simulink model "RoboticArm"  (R2023b)
settings: Solver=ode23t  StartTime=0.0  StopTime=100  RelTol=1e-3
model workspace: external: MATLAB File D:\Projects\RoboticArm\RoboticArm_DataFile1.m (data not in the file)
undefined symbols (not defined in the file or in its folder): dfdbk, dFilt, nfdbk, nFilt, smiData, ST, X, Y, Z
libraries: sm_lib x180, fl_lib x129, nesl_utility x69, ee_lib x39, slpidlib x25, simulink x18, SignalEditorBlockLib x1
(part 1 of 7)
settings Model: Creator=ASUS  LastModifiedBy=ASUS

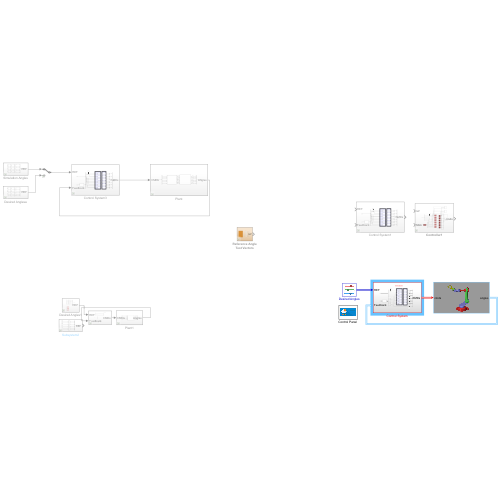
[thumbnail: Simulink's stored preview of the top-level diagram]
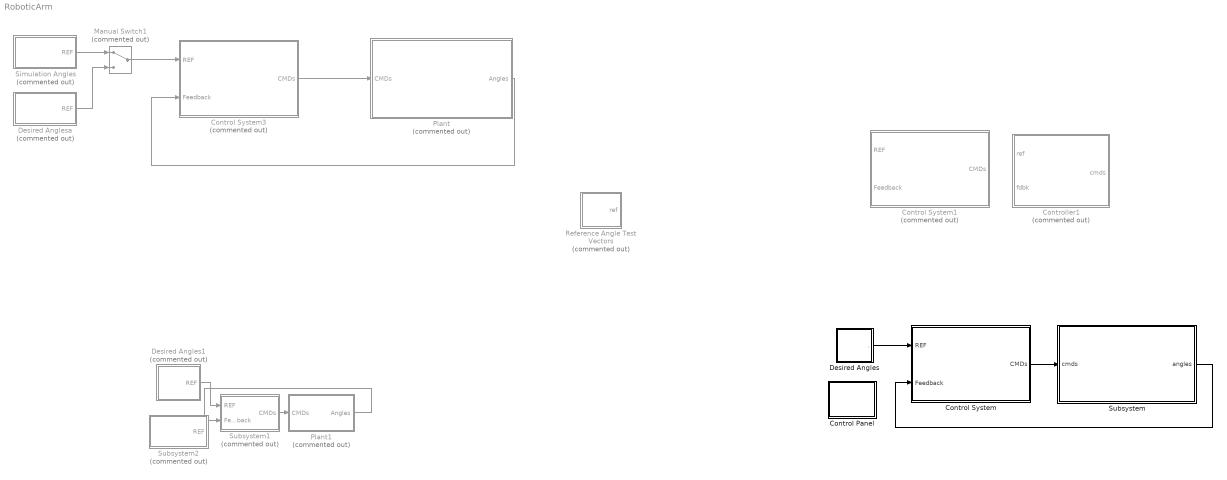
== system RoboticArm ==
  "Control Panel " : Subsystem
      mask Display: image('OIP (1).jpg');
  Control System : Subsystem
  Control System1 : Subsystem  Commented=on
  Control System3 : Subsystem  Commented=on
  Controller1 : Subsystem  Commented=on
  Desired Angles : Subsystem
      mask Display: image('reference.webp');
  Desired Angles1 : Subsystem  Commented=on
  Desired Anglesa : Subsystem  Commented=on
  Manual Switch1 : ManualSwitch  Commented=on
  Plant : Subsystem  Commented=on
  Plant1 : Subsystem  Commented=on
  Reference Angle Test Vectors : Subsystem  Commented=on
  Simulation Angles : Subsystem  Commented=on
  Subsystem : Subsystem
      mask Display: image('Screenshot 2024-04-15 220619.png');
  Subsystem1 : Subsystem  Commented=on
  Subsystem2 : Subsystem  Commented=on
  wires:
  Plant/1(Angles) -> Control System3/2(Feedback)
  Control System3/1(CMDs) -> Plant/1(CMDs)
  Subsystem1/1(CMDs) -> Plant1/1(CMDs)
  Plant1/1(Angles) -> Subsystem1/2(Feedback)
  Desired Angles1/1(REF) -> Subsystem1/1(REF)
  Desired Angles/1(.) -> Control System/1(REF)
  Subsystem/1(angles) -> Control System/2(Feedback)
  Control System/1(CMDs) -> Subsystem/1(cmds)
  Simulation Angles/1(REF) -> Manual Switch1/1
  Manual Switch1/1 -> Control System3/1(REF)
  Desired Anglesa/1(REF) -> Manual Switch1/2

== system RoboticArm/Control Panel  ==
  "Bicep " : Subsystem
      mask Display: image('Screenshot 2024-04-15 210704.png');
  Forearm : Subsystem
      mask Display: image('Screenshot 2024-04-15 210823.png');
  Gripper : Subsystem
      mask Display: image('Screenshot 2024-04-15 212833.png');
  Gripper base : Subsystem
      mask Display: image('Screenshot 2024-04-15 211030.png');
  Hand : Subsystem
      mask Display: image('Screenshot 2024-04-15 210946.png');
  Slider{,1..5} (6 alike) : SliderBlock  ScaleMin=-90  ScaleMax=90
  Slider6 : SliderBlock  ScaleMin=100  ScaleMax=140
  Turntable : Subsystem
      mask Display: image('Screenshot 2024-04-15 210633.png');
  Wrist : Subsystem
      mask Display: image('Screenshot 2024-04-15 210901.png');

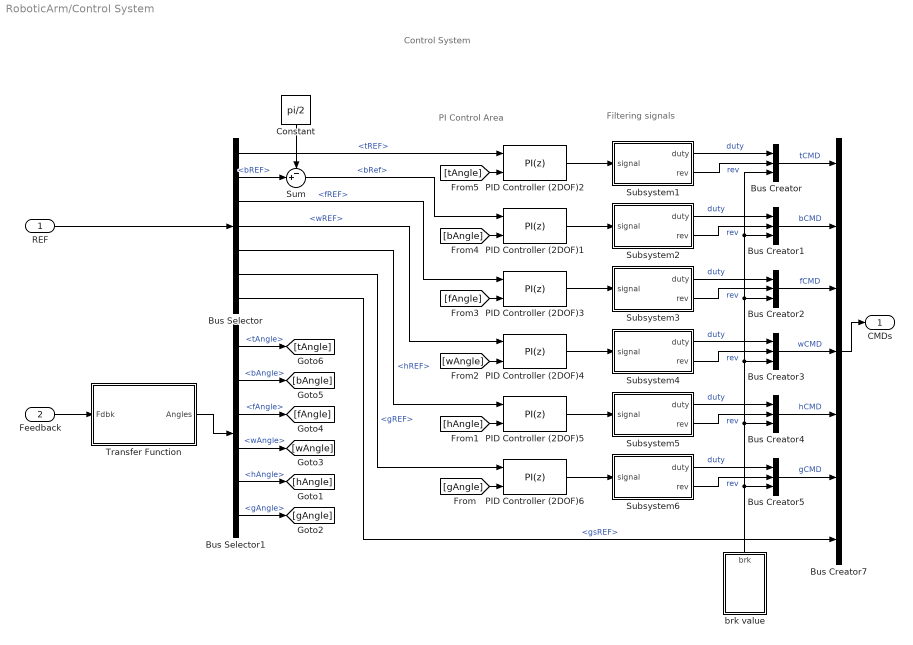
== system RoboticArm/Control System ==
  note: Control System
  note: PI Control Area
  note: Filtering signals
  REF : Inport
  Feedback : Inport  Port=2
  Bus Creator{,1..5} (6 alike) : BusCreator  Inputs=3
  Bus Creator7 : BusCreator  Inputs=7
  Bus Selector : BusSelector  OutputSignals=tREF,bREF,fREF,wREF,hREF,gREF,gsREF
  Bus Selector1 : BusSelector  OutputSignals=tAngle,bAngle,fAngle,wAngle,hAngle,gAngle
  Constant : Constant  Value=pi/2
  PID Controller (2DOF)1 : slpidlib/PID Controller (2DOF)  Controller=PI  Form=Parallel  TimeDomain=Discrete-time  UseExternalTs=off  SampleTime=ST  IntegratorMethod=Forward Euler  FilterMethod=Forward Euler  ControllerParametersSource=internal  P=6  I=3  UseKiTs=off  D=0.001  N=100  UseFilter=on  b=1  c=1  TunerSelectOption=Frequency Response Based  InitialConditionSource=internal  InitialConditionForIntegrator=0  InitialConditionForFilter=0  DifferentiatorICPrevScaledInput=0  ExternalReset=none  TrackingMode=off  Kt=1  LimitOutput=off  SatLimitsSource=internal  UpperSaturationLimit=inf  LowerSaturationLimit=-inf  LinearizeAsGain=on  AntiWindupMode=none  Kb=1  LimitIntegrator=off  UpperIntegratorSaturationLimit=inf  LowerIntegratorSaturationLimit=-inf  POutMin=[]  POutMax=[]  IOutMin=[]  IOutMax=[]  DOutMin=[]  DOutMax=[]  NOutMin=[]  NOutMax=[]  bOutMin=[]  bOutMax=[]  cOutMin=[]  cOutMax=[]  SumOutMin=[]  SumOutMax=[]  SaturationOutMin=[]  SaturationOutMax=[]  PParamMin=[]  PParamMax=[]  IParamMin=[]  IParamMax=[]  DParamMin=[]  DParamMax=[]  NParamMin=[]  NParamMax=[]  bParamMin=[]  bParamMax=[]  cParamMin=[]  cParamMax=[]  KbParamMin=[]  KbParamMax=[]  KtParamMin=[]  KtParamMax=[]  KbOutMin=[]  KbOutMax=[]  KtOutMin=[]  KtOutMax=[]  IntegratorOutMin=[]  IntegratorOutMax=[]  FilterOutMin=[]  FilterOutMax=[]  SumI1OutMin=[]  SumI1OutMax=[]  SumI2OutMin=[]  SumI2OutMax=[]  SumI3OutMin=[]  SumI3OutMax=[]  SumI4OutMin=[]  SumI4OutMax=[]  SumDOutMin=[]  SumDOutMax=[]  Sum1OutMin=[]  Sum1OutMax=[]  Sum2OutMin=[]  Sum2OutMax=[]  Sum3OutMin=[]  Sum3OutMax=[]  DifferentiatorOutMin=[]  DifferentiatorOutMax=[]  FilterDiffOutCoefMin=[]  FilterDiffOutCoefMax=[]  ReciprocalOutMin=[]  ReciprocalOutMax=[]  SumDenOutMin=[]  SumDenOutMax=[]  SumNumOutMin=[]  SumNumOutMax=[]  DivideOutMin=[]  DivideOutMax=[]  UdiffTsProdOutMin=[]  UdiffTsProdOutMax=[]  NTsProdOutMin=[]  NTsProdOutMax=[]  UintegralTsProdOutMin=[]  UintegralTsProdOutMax=[]  UngainTsProdOutMin=[]  UngainTsProdOutMax=[]  ClampingZeroOutDataTypeStr=Inherit: Inherit via back propagation  ClampingZeroOutMin=[]  ClampingZeroOutMax=[]  FilterDenConstantOutDataTypeStr=Inherit: Inherit via back propagation  FilterDenConstantOutMin=[]  FilterDenConstantOutMax=[]  PCopyOutDataTypeStr=Inherit: Inherit via back propagation  PCopyOutMin=[]  PCopyOutMax=[]  NCopyOutDataTypeStr=Inherit: Inherit via back propagation  NCopyOutMin=[]  NCopyOutMax=[]  IntegratorContinuousStateAttributes=''  IntegratorStateMustResolveToSignalObject=off  IntegratorRTWStateStorageClass=Auto  FilterContinuousStateAttributes=''  FilterStateMustResolveToSignalObject=off  FilterRTWStateStorageClass=Auto  ParallelPVariant=InternalParameters  IdealPVariant=Disabled  IVariant=InternalParameters  DVariant=Disabled  bVariant=InternalParameters  cVariant=Disabled  IntegratorVariant=Discrete  SatVariant=Disabled  AWVariant=Passthrough  PCopyVariant=Disabled  TRVariant=Disabled  FdbkBlocksVariant=Forward  IdealPFdbkVariant=Disabled  SatFdbkVariant=Disabled  DerivativeFilterVariant=Disabled  NVariant=Disabled  NCopyVariant=Disabled_SignalSpec  FilterICVariant=Disabled  IntegratorICVariant=InternalICs  ExternalResetVariant=Disabled  TRSumVariant=Passthrough  SumFdbkVariant=Disabled  SumVariant=Sum_PI  TsampFilterVariant=InternalTs  TsampNgainVariant=Passthrough  TsampIntegralVariant=Disabled_SignalSpec  ExternalSaturationOutDataTypeStr=Inherit: Same as second input
  PID Controller (2DOF){2,4..6} (4 alike) : slpidlib/PID Controller (2DOF)  Controller=PI  Form=Parallel  TimeDomain=Discrete-time  UseExternalTs=off  SampleTime=ST  IntegratorMethod=Forward Euler  FilterMethod=Forward Euler  ControllerParametersSource=internal  P=3  I=3  UseKiTs=off  D=0.001  N=100  UseFilter=on  b=1  c=1  TunerSelectOption=Frequency Response Based  InitialConditionSource=internal  InitialConditionForIntegrator=0  InitialConditionForFilter=0  DifferentiatorICPrevScaledInput=0  ExternalReset=none  TrackingMode=off  Kt=1  LimitOutput=off  SatLimitsSource=internal  UpperSaturationLimit=inf  LowerSaturationLimit=-inf  LinearizeAsGain=on  AntiWindupMode=none  Kb=1  LimitIntegrator=off  UpperIntegratorSaturationLimit=inf  LowerIntegratorSaturationLimit=-inf  POutMin=[]  POutMax=[]  IOutMin=[]  IOutMax=[]  DOutMin=[]  DOutMax=[]  NOutMin=[]  NOutMax=[]  bOutMin=[]  bOutMax=[]  cOutMin=[]  cOutMax=[]  SumOutMin=[]  SumOutMax=[]  SaturationOutMin=[]  SaturationOutMax=[]  PParamMin=[]  PParamMax=[]  IParamMin=[]  IParamMax=[]  DParamMin=[]  DParamMax=[]  NParamMin=[]  NParamMax=[]  bParamMin=[]  bParamMax=[]  cParamMin=[]  cParamMax=[]  KbParamMin=[]  KbParamMax=[]  KtParamMin=[]  KtParamMax=[]  KbOutMin=[]  KbOutMax=[]  KtOutMin=[]  KtOutMax=[]  IntegratorOutMin=[]  IntegratorOutMax=[]  FilterOutMin=[]  FilterOutMax=[]  SumI1OutMin=[]  SumI1OutMax=[]  SumI2OutMin=[]  SumI2OutMax=[]  SumI3OutMin=[]  SumI3OutMax=[]  SumI4OutMin=[]  SumI4OutMax=[]  SumDOutMin=[]  SumDOutMax=[]  Sum1OutMin=[]  Sum1OutMax=[]  Sum2OutMin=[]  Sum2OutMax=[]  Sum3OutMin=[]  Sum3OutMax=[]  DifferentiatorOutMin=[]  DifferentiatorOutMax=[]  FilterDiffOutCoefMin=[]  FilterDiffOutCoefMax=[]  ReciprocalOutMin=[]  ReciprocalOutMax=[]  SumDenOutMin=[]  SumDenOutMax=[]  SumNumOutMin=[]  SumNumOutMax=[]  DivideOutMin=[]  DivideOutMax=[]  UdiffTsProdOutMin=[]  UdiffTsProdOutMax=[]  NTsProdOutMin=[]  NTsProdOutMax=[]  UintegralTsProdOutMin=[]  UintegralTsProdOutMax=[]  UngainTsProdOutMin=[]  UngainTsProdOutMax=[]  ClampingZeroOutDataTypeStr=Inherit: Inherit via back propagation  ClampingZeroOutMin=[]  ClampingZeroOutMax=[]  FilterDenConstantOutDataTypeStr=Inherit: Inherit via back propagation  FilterDenConstantOutMin=[]  FilterDenConstantOutMax=[]  PCopyOutDataTypeStr=Inherit: Inherit via back propagation  PCopyOutMin=[]  PCopyOutMax=[]  NCopyOutDataTypeStr=Inherit: Inherit via back propagation  NCopyOutMin=[]  NCopyOutMax=[]  IntegratorContinuousStateAttributes=''  IntegratorStateMustResolveToSignalObject=off  IntegratorRTWStateStorageClass=Auto  FilterContinuousStateAttributes=''  FilterStateMustResolveToSignalObject=off  FilterRTWStateStorageClass=Auto  ParallelPVariant=InternalParameters  IdealPVariant=Disabled  IVariant=InternalParameters  DVariant=Disabled  bVariant=InternalParameters  cVariant=Disabled  IntegratorVariant=Discrete  SatVariant=Disabled  AWVariant=Passthrough  PCopyVariant=Disabled  TRVariant=Disabled  FdbkBlocksVariant=Forward  IdealPFdbkVariant=Disabled  SatFdbkVariant=Disabled  DerivativeFilterVariant=Disabled  NVariant=Disabled  NCopyVariant=Disabled_SignalSpec  FilterICVariant=Disabled  IntegratorICVariant=InternalICs  ExternalResetVariant=Disabled  TRSumVariant=Passthrough  SumFdbkVariant=Disabled  SumVariant=Sum_PI  TsampFilterVariant=InternalTs  TsampNgainVariant=Passthrough  TsampIntegralVariant=Disabled_SignalSpec  ExternalSaturationOutDataTypeStr=Inherit: Same as second input
  PID Controller (2DOF)3 : slpidlib/PID Controller (2DOF)  Controller=PI  Form=Parallel  TimeDomain=Discrete-time  UseExternalTs=off  SampleTime=ST  IntegratorMethod=Forward Euler  FilterMethod=Forward Euler  ControllerParametersSource=internal  P=6  I=3  UseKiTs=off  D=0.001  N=100  UseFilter=on  b=1  c=1  TunerSelectOption=Frequency Response Based  InitialConditionSource=internal  InitialConditionForIntegrator=0  InitialConditionForFilter=0  DifferentiatorICPrevScaledInput=0  ExternalReset=none  TrackingMode=off  Kt=1  LimitOutput=off  SatLimitsSource=internal  UpperSaturationLimit=inf  LowerSaturationLimit=-inf  LinearizeAsGain=on  AntiWindupMode=none  Kb=1  LimitIntegrator=off  UpperIntegratorSaturationLimit=inf  LowerIntegratorSaturationLimit=-inf  POutMin=[]  POutMax=[]  IOutMin=[]  IOutMax=[]  DOutMin=[]  DOutMax=[]  NOutMin=[]  NOutMax=[]  bOutMin=[]  bOutMax=[]  cOutMin=[]  cOutMax=[]  SumOutMin=[]  SumOutMax=[]  SaturationOutMin=[]  SaturationOutMax=[]  PParamMin=[]  PParamMax=[]  IParamMin=[]  IParamMax=[]  DParamMin=[]  DParamMax=[]  NParamMin=[]  NParamMax=[]  bParamMin=[]  bParamMax=[]  cParamMin=[]  cParamMax=[]  KbParamMin=[]  KbParamMax=[]  KtParamMin=[]  KtParamMax=[]  KbOutMin=[]  KbOutMax=[]  KtOutMin=[]  KtOutMax=[]  IntegratorOutMin=[]  IntegratorOutMax=[]  FilterOutMin=[]  FilterOutMax=[]  SumI1OutMin=[]  SumI1OutMax=[]  SumI2OutMin=[]  SumI2OutMax=[]  SumI3OutMin=[]  SumI3OutMax=[]  SumI4OutMin=[]  SumI4OutMax=[]  SumDOutMin=[]  SumDOutMax=[]  Sum1OutMin=[]  Sum1OutMax=[]  Sum2OutMin=[]  Sum2OutMax=[]  Sum3OutMin=[]  Sum3OutMax=[]  DifferentiatorOutMin=[]  DifferentiatorOutMax=[]  FilterDiffOutCoefMin=[]  FilterDiffOutCoefMax=[]  ReciprocalOutMin=[]  ReciprocalOutMax=[]  SumDenOutMin=[]  SumDenOutMax=[]  SumNumOutMin=[]  SumNumOutMax=[]  DivideOutMin=[]  DivideOutMax=[]  UdiffTsProdOutMin=[]  UdiffTsProdOutMax=[]  NTsProdOutMin=[]  NTsProdOutMax=[]  UintegralTsProdOutMin=[]  UintegralTsProdOutMax=[]  UngainTsProdOutMin=[]  UngainTsProdOutMax=[]  ClampingZeroOutDataTypeStr=Inherit: Inherit via back propagation  ClampingZeroOutMin=[]  ClampingZeroOutMax=[]  FilterDenConstantOutDataTypeStr=Inherit: Inherit via back propagation  FilterDenConstantOutMin=[]  FilterDenConstantOutMax=[]  PCopyOutDataTypeStr=Inherit: Inherit via back propagation  PCopyOutMin=[]  PCopyOutMax=[]  NCopyOutDataTypeStr=Inherit: Inherit via back propagation  NCopyOutMin=[]  NCopyOutMax=[]  IntegratorContinuousStateAttributes=''  IntegratorStateMustResolveToSignalObject=off  IntegratorRTWStateStorageClass=Auto  FilterContinuousStateAttributes=''  FilterStateMustResolveToSignalObject=off  FilterRTWStateStorageClass=Auto  ParallelPVariant=InternalParameters  IdealPVariant=Disabled  IVariant=InternalParameters  DVariant=Disabled  bVariant=InternalParameters  cVariant=Disabled  IntegratorVariant=Discrete  SatVariant=Disabled  AWVariant=Passthrough  PCopyVariant=Disabled  TRVariant=Disabled  FdbkBlocksVariant=Forward  IdealPFdbkVariant=Disabled  SatFdbkVariant=Disabled  DerivativeFilterVariant=Disabled  NVariant=Disabled  NCopyVariant=Disabled_SignalSpec  FilterICVariant=Disabled  IntegratorICVariant=InternalICs  ExternalResetVariant=Disabled  TRSumVariant=Passthrough  SumFdbkVariant=Disabled  SumVariant=Sum_PI  TsampFilterVariant=InternalTs  TsampNgainVariant=Passthrough  TsampIntegralVariant=Disabled_SignalSpec  ExternalSaturationOutDataTypeStr=Inherit: Same as second input
  Subsystem1 : Subsystem
  Subsystem2 : Subsystem
  Subsystem3 : Subsystem
  Subsystem4 : Subsystem
  Subsystem5 : Subsystem
  Subsystem6 : Subsystem
  Sum : Sum  Inputs=-+|
  Transfer Function : Subsystem
  brk value : Subsystem
  CMDs : Outport
  wires:
  Subsystem3/2(rev) -> Bus Creator2/2  "rev"
  Subsystem2/1(duty) -> Bus Creator1/1  "duty"
  REF/1 -> Bus Selector/1
  Bus Creator1/1 -> Bus Creator7/2  "bCMD"
  Subsystem1/1(duty) -> Bus Creator/1  "duty"
  Subsystem3/1(duty) -> Bus Creator2/1  "duty"
  Bus Creator3/1 -> Bus Creator7/4  "wCMD"
  Subsystem1/2(rev) -> Bus Creator/2  "rev"
  Subsystem6/1(duty) -> Bus Creator5/1  "duty"
  Subsystem6/2(rev) -> Bus Creator5/2  "rev"
  Bus Creator7/1 -> CMDs/1
  Bus Creator2/1 -> Bus Creator7/3  "fCMD"
  Subsystem2/2(rev) -> Bus Creator1/2  "rev"
  Subsystem4/2(rev) -> Bus Creator3/2  "rev"
  Bus Creator/1 -> Bus Creator7/1  "tCMD"
  Subsystem4/1(duty) -> Bus Creator3/1  "duty"
  Subsystem5/1(duty) -> Bus Creator4/1  "duty"
  Subsystem5/2(rev) -> Bus Creator4/2  "rev"
  Bus Creator5/1 -> Bus Creator7/6  "gCMD"
  Bus Creator4/1 -> Bus Creator7/5  "hCMD"
  Bus Selector/2 -> Sum/2  "<bREF>"
  Constant/1 -> Sum/1
  Feedback/1 -> Transfer Function/1(Fdbk)
  Transfer Function/1(Angles) -> Bus Selector1/1
  PID Controller (2DOF)2/1 -> Subsystem1/1(signal)
  Bus Selector/1 -> PID Controller (2DOF)2/1  "<tREF>"
  PID Controller (2DOF)1/1 -> Subsystem2/1(signal)
  PID Controller (2DOF)3/1 -> Subsystem3/1(signal)
  PID Controller (2DOF)4/1 -> Subsystem4/1(signal)
  PID Controller (2DOF)5/1 -> Subsystem5/1(signal)
  PID Controller (2DOF)6/1 -> Subsystem6/1(signal)
  Sum/1 -> PID Controller (2DOF)1/1  "<bRef>"
  Bus Selector/3 -> PID Controller (2DOF)3/1  "<fREF>"
  Bus Selector/4 -> PID Controller (2DOF)4/1  "<wREF>"
  Bus Selector/5 -> PID Controller (2DOF)5/1  "<hREF>"
  Bus Selector/6 -> PID Controller (2DOF)6/1  "<gREF>"
  Bus Selector/7 -> Bus Creator7/7  "<gsREF>"
  brk value/1(brk) -> Bus Creator5/3, Bus Creator4/3, Bus Creator3/3, Bus Creator2/3, Bus Creator1/3, Bus Creator/3
  Bus Selector1/6 -> [gAngle]  "<gAngle>"
  [gAngle] -> PID Controller (2DOF)6/2
  Bus Selector1/5 -> [hAngle]  "<hAngle>"
  Bus Selector1/4 -> [wAngle]  "<wAngle>"
  Bus Selector1/3 -> [fAngle]  "<fAngle>"
  Bus Selector1/2 -> [bAngle]  "<bAngle>"
  Bus Selector1/1 -> [tAngle]  "<tAngle>"
  [hAngle] -> PID Controller (2DOF)5/2
  [wAngle] -> PID Controller (2DOF)4/2
  [fAngle] -> PID Controller (2DOF)3/2
  [bAngle] -> PID Controller (2DOF)1/2
  [tAngle] -> PID Controller (2DOF)2/2

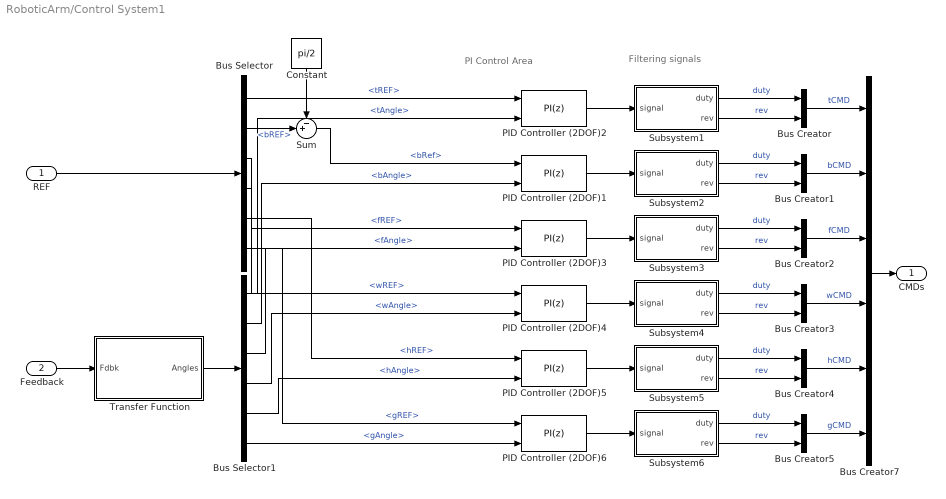
== system RoboticArm/Control System1 ==
  note: Filtering signals
  note: PI Control Area
  REF : Inport
  Feedback : Inport  Port=2
  Bus Creator{,1..5} (6 alike) : BusCreator  Inputs=2
  Bus Creator7 : BusCreator  Inputs=6
  Bus Selector : BusSelector  OutputSignals=tREF,bREF,fREF,wREF,hREF,gREF
  Bus Selector1 : BusSelector  OutputSignals=tAngle,bAngle,fAngle,wAngle,hAngle,gAngle
  Constant : Constant  Value=pi/2
  PID Controller (2DOF){1..6} (6 alike) : slpidlib/PID Controller (2DOF)  Controller=PI  Form=Parallel  TimeDomain=Discrete-time  UseExternalTs=off  SampleTime=ST  IntegratorMethod=Forward Euler  FilterMethod=Forward Euler  ControllerParametersSource=internal  P=3  I=3  UseKiTs=off  D=0.001  N=100  UseFilter=on  b=1  c=1  TunerSelectOption=Frequency Response Based  InitialConditionSource=internal  InitialConditionForIntegrator=0  InitialConditionForFilter=0  DifferentiatorICPrevScaledInput=0  ExternalReset=none  TrackingMode=off  Kt=1  LimitOutput=off  SatLimitsSource=internal  UpperSaturationLimit=inf  LowerSaturationLimit=-inf  LinearizeAsGain=on  AntiWindupMode=none  Kb=1  LimitIntegrator=off  UpperIntegratorSaturationLimit=inf  LowerIntegratorSaturationLimit=-inf  POutMin=[]  POutMax=[]  IOutMin=[]  IOutMax=[]  DOutMin=[]  DOutMax=[]  NOutMin=[]  NOutMax=[]  bOutMin=[]  bOutMax=[]  cOutMin=[]  cOutMax=[]  SumOutMin=[]  SumOutMax=[]  SaturationOutMin=[]  SaturationOutMax=[]  PParamMin=[]  PParamMax=[]  IParamMin=[]  IParamMax=[]  DParamMin=[]  DParamMax=[]  NParamMin=[]  NParamMax=[]  bParamMin=[]  bParamMax=[]  cParamMin=[]  cParamMax=[]  KbParamMin=[]  KbParamMax=[]  KtParamMin=[]  KtParamMax=[]  KbOutMin=[]  KbOutMax=[]  KtOutMin=[]  KtOutMax=[]  IntegratorOutMin=[]  IntegratorOutMax=[]  FilterOutMin=[]  FilterOutMax=[]  SumI1OutMin=[]  SumI1OutMax=[]  SumI2OutMin=[]  SumI2OutMax=[]  SumI3OutMin=[]  SumI3OutMax=[]  SumI4OutMin=[]  SumI4OutMax=[]  SumDOutMin=[]  SumDOutMax=[]  Sum1OutMin=[]  Sum1OutMax=[]  Sum2OutMin=[]  Sum2OutMax=[]  Sum3OutMin=[]  Sum3OutMax=[]  DifferentiatorOutMin=[]  DifferentiatorOutMax=[]  FilterDiffOutCoefMin=[]  FilterDiffOutCoefMax=[]  ReciprocalOutMin=[]  ReciprocalOutMax=[]  SumDenOutMin=[]  SumDenOutMax=[]  SumNumOutMin=[]  SumNumOutMax=[]  DivideOutMin=[]  DivideOutMax=[]  UdiffTsProdOutMin=[]  UdiffTsProdOutMax=[]  NTsProdOutMin=[]  NTsProdOutMax=[]  UintegralTsProdOutMin=[]  UintegralTsProdOutMax=[]  UngainTsProdOutMin=[]  UngainTsProdOutMax=[]  ClampingZeroOutDataTypeStr=Inherit: Inherit via back propagation  ClampingZeroOutMin=[]  ClampingZeroOutMax=[]  FilterDenConstantOutDataTypeStr=Inherit: Inherit via back propagation  FilterDenConstantOutMin=[]  FilterDenConstantOutMax=[]  PCopyOutDataTypeStr=Inherit: Inherit via back propagation  PCopyOutMin=[]  PCopyOutMax=[]  NCopyOutDataTypeStr=Inherit: Inherit via back propagation  NCopyOutMin=[]  NCopyOutMax=[]  IntegratorContinuousStateAttributes=''  IntegratorStateMustResolveToSignalObject=off  IntegratorRTWStateStorageClass=Auto  FilterContinuousStateAttributes=''  FilterStateMustResolveToSignalObject=off  FilterRTWStateStorageClass=Auto  ParallelPVariant=InternalParameters  IdealPVariant=Disabled  IVariant=InternalParameters  DVariant=Disabled  bVariant=InternalParameters  cVariant=Disabled  IntegratorVariant=Discrete  SatVariant=Disabled  AWVariant=Passthrough  PCopyVariant=Disabled  TRVariant=Disabled  FdbkBlocksVariant=Forward  IdealPFdbkVariant=Disabled  SatFdbkVariant=Disabled  DerivativeFilterVariant=Disabled  NVariant=Disabled  NCopyVariant=Disabled_SignalSpec  FilterICVariant=Disabled  IntegratorICVariant=InternalICs  ExternalResetVariant=Disabled  TRSumVariant=Passthrough  SumFdbkVariant=Disabled  SumVariant=Sum_PI  TsampFilterVariant=InternalTs  TsampNgainVariant=Passthrough  TsampIntegralVariant=Disabled_SignalSpec  ExternalSaturationOutDataTypeStr=Inherit: Same as second input
  Subsystem1 : Subsystem
  Subsystem2 : Subsystem
  Subsystem3 : Subsystem
  Subsystem4 : Subsystem
  Subsystem5 : Subsystem
  Subsystem6 : Subsystem
  Sum : Sum  Inputs=-+|
  Transfer Function : Subsystem
  CMDs : Outport
  wires:
  Bus Selector1/6 -> PID Controller (2DOF)6/2  "<gAngle>"
  Bus Selector1/5 -> PID Controller (2DOF)5/2  "<hAngle>"
  Bus Selector1/4 -> PID Controller (2DOF)4/2  "<wAngle>"
  Bus Selector1/3 -> PID Controller (2DOF)3/2  "<fAngle>"
  Bus Selector1/2 -> PID Controller (2DOF)1/2  "<bAngle>"
  Bus Selector1/1 -> PID Controller (2DOF)2/2  "<tAngle>"
  Bus Selector/6 -> PID Controller (2DOF)6/1  "<gREF>"
  Bus Selector/5 -> PID Controller (2DOF)5/1  "<hREF>"
  Bus Selector/4 -> PID Controller (2DOF)4/1  "<wREF>"
  Bus Selector/3 -> PID Controller (2DOF)3/1  "<fREF>"
  Sum/1 -> PID Controller (2DOF)1/1  "<bRef>"
  PID Controller (2DOF)6/1 -> Subsystem6/1(signal)
  PID Controller (2DOF)5/1 -> Subsystem5/1(signal)
  PID Controller (2DOF)4/1 -> Subsystem4/1(signal)
  PID Controller (2DOF)3/1 -> Subsystem3/1(signal)
  PID Controller (2DOF)1/1 -> Subsystem2/1(signal)
  Bus Selector/1 -> PID Controller (2DOF)2/1  "<tREF>"
  PID Controller (2DOF)2/1 -> Subsystem1/1(signal)
  Transfer Function/1(Angles) -> Bus Selector1/1
  Feedback/1 -> Transfer Function/1(Fdbk)
  Constant/1 -> Sum/1
  Bus Selector/2 -> Sum/2  "<bREF>"
  Bus Creator4/1 -> Bus Creator7/5  "hCMD"
  Bus Creator5/1 -> Bus Creator7/6  "gCMD"
  Subsystem5/2(rev) -> Bus Creator4/2  "rev"
  Subsystem5/1(duty) -> Bus Creator4/1  "duty"
  Subsystem4/1(duty) -> Bus Creator3/1  "duty"
  Bus Creator/1 -> Bus Creator7/1  "tCMD"
  Subsystem4/2(rev) -> Bus Creator3/2  "rev"
  Subsystem2/2(rev) -> Bus Creator1/2  "rev"
  Bus Creator2/1 -> Bus Creator7/3  "fCMD"
  Bus Creator7/1 -> CMDs/1
  Subsystem6/2(rev) -> Bus Creator5/2  "rev"
  Subsystem6/1(duty) -> Bus Creator5/1  "duty"
  Subsystem1/2(rev) -> Bus Creator/2  "rev"
  Bus Creator3/1 -> Bus Creator7/4  "wCMD"
  Subsystem3/1(duty) -> Bus Creator2/1  "duty"
  Subsystem1/1(duty) -> Bus Creator/1  "duty"
  Bus Creator1/1 -> Bus Creator7/2  "bCMD"
  REF/1 -> Bus Selector/1
  Subsystem2/1(duty) -> Bus Creator1/1  "duty"
  Subsystem3/2(rev) -> Bus Creator2/2  "rev"

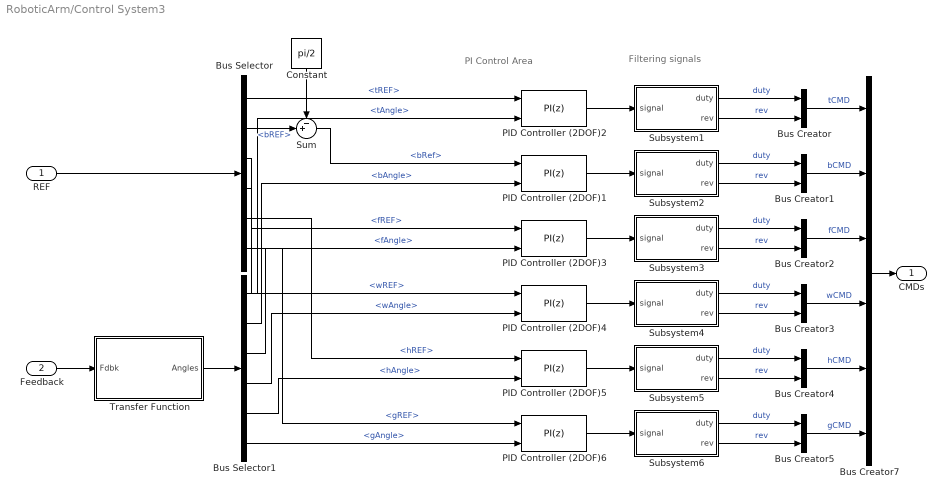
== system RoboticArm/Control System3 ==
  note: PI Control Area
  note: Filtering signals
  REF : Inport
  Feedback : Inport  Port=2
  Bus Creator{,1..5} (6 alike) : BusCreator  Inputs=2
  Bus Creator7 : BusCreator  Inputs=6
  Bus Selector : BusSelector  OutputSignals=tREF,bREF,fREF,wREF,hREF,gREF
  Bus Selector1 : BusSelector  OutputSignals=tAngle,bAngle,fAngle,wAngle,hAngle,gAngle
  Constant : Constant  Value=pi/2
  PID Controller (2DOF){1..6} (6 alike) : slpidlib/PID Controller (2DOF)  Controller=PI  Form=Parallel  TimeDomain=Discrete-time  UseExternalTs=off  SampleTime=ST  IntegratorMethod=Forward Euler  FilterMethod=Forward Euler  ControllerParametersSource=internal  P=3  I=3  UseKiTs=off  D=0.001  N=100  UseFilter=on  b=1  c=1  TunerSelectOption=Frequency Response Based  InitialConditionSource=internal  InitialConditionForIntegrator=0  InitialConditionForFilter=0  DifferentiatorICPrevScaledInput=0  ExternalReset=none  TrackingMode=off  Kt=1  LimitOutput=off  SatLimitsSource=internal  UpperSaturationLimit=inf  LowerSaturationLimit=-inf  LinearizeAsGain=on  AntiWindupMode=none  Kb=1  LimitIntegrator=off  UpperIntegratorSaturationLimit=inf  LowerIntegratorSaturationLimit=-inf  POutMin=[]  POutMax=[]  IOutMin=[]  IOutMax=[]  DOutMin=[]  DOutMax=[]  NOutMin=[]  NOutMax=[]  bOutMin=[]  bOutMax=[]  cOutMin=[]  cOutMax=[]  SumOutMin=[]  SumOutMax=[]  SaturationOutMin=[]  SaturationOutMax=[]  PParamMin=[]  PParamMax=[]  IParamMin=[]  IParamMax=[]  DParamMin=[]  DParamMax=[]  NParamMin=[]  NParamMax=[]  bParamMin=[]  bParamMax=[]  cParamMin=[]  cParamMax=[]  KbParamMin=[]  KbParamMax=[]  KtParamMin=[]  KtParamMax=[]  KbOutMin=[]  KbOutMax=[]  KtOutMin=[]  KtOutMax=[]  IntegratorOutMin=[]  IntegratorOutMax=[]  FilterOutMin=[]  FilterOutMax=[]  SumI1OutMin=[]  SumI1OutMax=[]  SumI2OutMin=[]  SumI2OutMax=[]  SumI3OutMin=[]  SumI3OutMax=[]  SumI4OutMin=[]  SumI4OutMax=[]  SumDOutMin=[]  SumDOutMax=[]  Sum1OutMin=[]  Sum1OutMax=[]  Sum2OutMin=[]  Sum2OutMax=[]  Sum3OutMin=[]  Sum3OutMax=[]  DifferentiatorOutMin=[]  DifferentiatorOutMax=[]  FilterDiffOutCoefMin=[]  FilterDiffOutCoefMax=[]  ReciprocalOutMin=[]  ReciprocalOutMax=[]  SumDenOutMin=[]  SumDenOutMax=[]  SumNumOutMin=[]  SumNumOutMax=[]  DivideOutMin=[]  DivideOutMax=[]  UdiffTsProdOutMin=[]  UdiffTsProdOutMax=[]  NTsProdOutMin=[]  NTsProdOutMax=[]  UintegralTsProdOutMin=[]  UintegralTsProdOutMax=[]  UngainTsProdOutMin=[]  UngainTsProdOutMax=[]  ClampingZeroOutDataTypeStr=Inherit: Inherit via back propagation  ClampingZeroOutMin=[]  ClampingZeroOutMax=[]  FilterDenConstantOutDataTypeStr=Inherit: Inherit via back propagation  FilterDenConstantOutMin=[]  FilterDenConstantOutMax=[]  PCopyOutDataTypeStr=Inherit: Inherit via back propagation  PCopyOutMin=[]  PCopyOutMax=[]  NCopyOutDataTypeStr=Inherit: Inherit via back propagation  NCopyOutMin=[]  NCopyOutMax=[]  IntegratorContinuousStateAttributes=''  IntegratorStateMustResolveToSignalObject=off  IntegratorRTWStateStorageClass=Auto  FilterContinuousStateAttributes=''  FilterStateMustResolveToSignalObject=off  FilterRTWStateStorageClass=Auto  ParallelPVariant=InternalParameters  IdealPVariant=Disabled  IVariant=InternalParameters  DVariant=Disabled  bVariant=InternalParameters  cVariant=Disabled  IntegratorVariant=Discrete  SatVariant=Disabled  AWVariant=Passthrough  PCopyVariant=Disabled  TRVariant=Disabled  FdbkBlocksVariant=Forward  IdealPFdbkVariant=Disabled  SatFdbkVariant=Disabled  DerivativeFilterVariant=Disabled  NVariant=Disabled  NCopyVariant=Disabled_SignalSpec  FilterICVariant=Disabled  IntegratorICVariant=InternalICs  ExternalResetVariant=Disabled  TRSumVariant=Passthrough  SumFdbkVariant=Disabled  SumVariant=Sum_PI  TsampFilterVariant=InternalTs  TsampNgainVariant=Passthrough  TsampIntegralVariant=Disabled_SignalSpec  ExternalSaturationOutDataTypeStr=Inherit: Same as second input
  Subsystem1 : Subsystem
  Subsystem2 : Subsystem
  Subsystem3 : Subsystem
  Subsystem4 : Subsystem
  Subsystem5 : Subsystem
  Subsystem6 : Subsystem
  Sum : Sum  Inputs=-+|
  Transfer Function : Subsystem
  CMDs : Outport
  wires:
  Subsystem3/2(rev) -> Bus Creator2/2  "rev"
  Subsystem2/1(duty) -> Bus Creator1/1  "duty"
  REF/1 -> Bus Selector/1
  Bus Creator1/1 -> Bus Creator7/2  "bCMD"
  Subsystem1/1(duty) -> Bus Creator/1  "duty"
  Subsystem3/1(duty) -> Bus Creator2/1  "duty"
  Bus Creator3/1 -> Bus Creator7/4  "wCMD"
  Subsystem1/2(rev) -> Bus Creator/2  "rev"
  Subsystem6/1(duty) -> Bus Creator5/1  "duty"
  Subsystem6/2(rev) -> Bus Creator5/2  "rev"
  Bus Creator7/1 -> CMDs/1
  Bus Creator2/1 -> Bus Creator7/3  "fCMD"
  Subsystem2/2(rev) -> Bus Creator1/2  "rev"
  Subsystem4/2(rev) -> Bus Creator3/2  "rev"
  Bus Creator/1 -> Bus Creator7/1  "tCMD"
  Subsystem4/1(duty) -> Bus Creator3/1  "duty"
  Subsystem5/1(duty) -> Bus Creator4/1  "duty"
  Subsystem5/2(rev) -> Bus Creator4/2  "rev"
  Bus Creator5/1 -> Bus Creator7/6  "gCMD"
  Bus Creator4/1 -> Bus Creator7/5  "hCMD"
  Bus Selector/2 -> Sum/2  "<bREF>"
  Constant/1 -> Sum/1
  Feedback/1 -> Transfer Function/1(Fdbk)
  Transfer Function/1(Angles) -> Bus Selector1/1
  PID Controller (2DOF)2/1 -> Subsystem1/1(signal)
  Bus Selector/1 -> PID Controller (2DOF)2/1  "<tREF>"
  PID Controller (2DOF)1/1 -> Subsystem2/1(signal)
  PID Controller (2DOF)3/1 -> Subsystem3/1(signal)
  PID Controller (2DOF)4/1 -> Subsystem4/1(signal)
  PID Controller (2DOF)5/1 -> Subsystem5/1(signal)
  PID Controller (2DOF)6/1 -> Subsystem6/1(signal)
  Sum/1 -> PID Controller (2DOF)1/1  "<bRef>"
  Bus Selector/3 -> PID Controller (2DOF)3/1  "<fREF>"
  Bus Selector/4 -> PID Controller (2DOF)4/1  "<wREF>"
  Bus Selector/5 -> PID Controller (2DOF)5/1  "<hREF>"
  Bus Selector/6 -> PID Controller (2DOF)6/1  "<gREF>"
  Bus Selector1/1 -> PID Controller (2DOF)2/2  "<tAngle>"
  Bus Selector1/2 -> PID Controller (2DOF)1/2  "<bAngle>"
  Bus Selector1/3 -> PID Controller (2DOF)3/2  "<fAngle>"
  Bus Selector1/4 -> PID Controller (2DOF)4/2  "<wAngle>"
  Bus Selector1/5 -> PID Controller (2DOF)5/2  "<hAngle>"
  Bus Selector1/6 -> PID Controller (2DOF)6/2  "<gAngle>"
